simulink model "Classical_vs_Segm_IaF"  (R2020b)
settings: Solver=VariableStepAuto  StartTime=0.0  StopTime=0.4  RelTol=1e-3
libraries: NeuroModelerLibrary x5
settings Model: Creator=Александра  LastModifiedBy=Александра

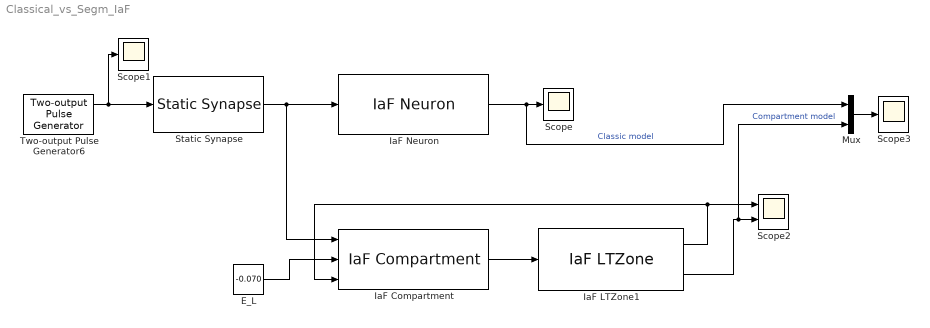
== system Classical_vs_Segm_IaF ==
  E_L : Constant  Value=-0.070
  IaF Compartment : NeuroModelerLibrary/Neuron Elements/IaF Compartment  tau_m=0.01  Cm=250e-12  I_const=0  E_L=-0.070  V_reset=-0.10  V_th=-0.055
  IaF LTZone1 : NeuroModelerLibrary/Neuron Elements/IaF LTZone  tau_m=0.01  Cm=250e-12  I_const=0  E_L=-0.070  V_reset=-0.10  V_th=-0.055
  IaF Neuron : NeuroModelerLibrary/Classic Models/IaF Neuron  tau_m=0.01  Cm=250e-12  I_const=0  E_L=-0.070  V_reset=-0.10  V_th=-0.055
  Mux : Mux  Inputs=2
  Scope : Scope
  Scope1 : Scope
  Scope2 : Scope  NumInputPorts=2
  Scope3 : Scope
  Static Synapse : NeuroModelerLibrary/Classic Models/Static Synapse  tau_syn=2e-3  I_syn=1e-8  weight=1  delay=1e-3
  Two-output Pulse Generator6 : NeuroModelerLibrary/Support/Two-output Pulse Generator  A=1  P1=200  P2=200  PW=1  ST=0.001  OOn1=0.1  OOff1=1.0  OOn2=0.1  OOff2=0.2
  wires:
  Static Synapse/1 -> IaF Compartment/1, IaF Neuron/1
  IaF Neuron/1 -> Mux/1, Scope/1  "Classic model"
  Two-output Pulse Generator6/1 -> Static Synapse/1, Scope1/1
  E_L/1 -> IaF Compartment/2
  IaF Compartment/1 -> IaF LTZone1/1
  IaF LTZone1/1 -> IaF Compartment/3, Scope2/1
  IaF LTZone1/2 -> Mux/2, Scope2/2  "Compartment model"
  Mux/1 -> Scope3/1
